simulink model "current_controller_AC"  (R2022a)
settings: Solver=FixedStepAuto  StartTime=0.0  StopTime=0.6  FixedStep=3e-8  RelTol=1e-3
values from neighbouring files (symbols this model uses):
  fs = 50*10^3    (= 50000)    [current_controller_parameters.m]
  Kii = 0.0307    [current_controller_parameters.m]
  Kpi = 9.65    [current_controller_parameters.m]
libraries: spsCurrentMeasurementLib x5, spsMosfetLib x4, spsVoltageMeasurementLib x4, spsSeriesRLCBranchLib x3, spsDCVoltageSourceLib x2, simulink x1, spsACVoltageSourceLib x1, spspowerguiLib x1
settings Model: Creator=RTX  LastModifiedBy=RTX

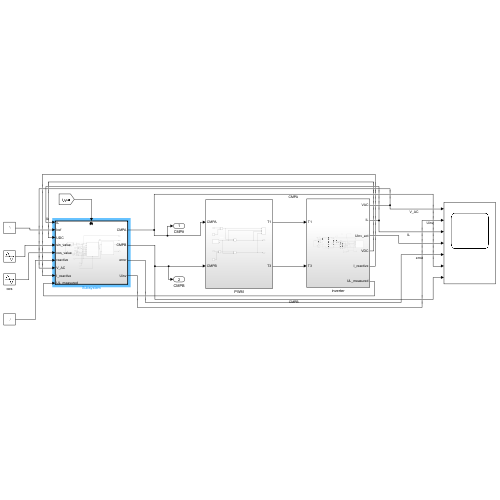
[thumbnail: Simulink's stored preview of the top-level diagram]
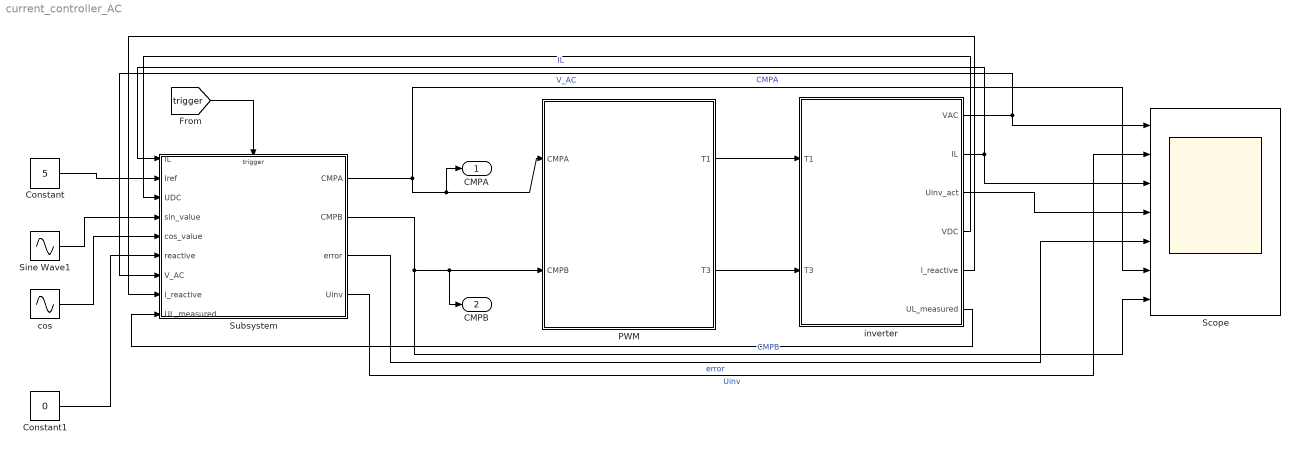
== system current_controller_AC ==
  Constant : Constant  Value=5
  Constant1 : Constant  Value=0
  PWM : Subsystem
  Scope : Scope  NumInputPorts=7
  Sine Wave1 : Sin  Frequency=2*pi*50  SampleTime=0
  Subsystem : Subsystem
  cos : Sin  Frequency=2*pi*50  Phase=pi/2  SampleTime=0
  inverter : Subsystem
  CMPA : Outport
  CMPB : Outport  Port=2
  wires:
  PWM/2(T3) -> inverter/2(T3)
  Subsystem/1(CMPA) -> Scope/6, CMPA/1, PWM/1(CMPA)  "CMPA"
  Constant/1 -> Subsystem/2(Iref)
  [trigger] -> Subsystem/Trigger
  inverter/2(IL) -> Scope/3, Subsystem/1(IL)  "IL"
  inverter/4(VDC) -> Subsystem/3(UDC)
  Sine Wave1/1 -> Subsystem/4(sin_value)
  cos/1 -> Subsystem/5(cos_value)
  Subsystem/2(CMPB) -> Scope/7, CMPB/1, PWM/2(CMPB)  "CMPB"
  PWM/1(T1) -> inverter/1(T1)
  Subsystem/3(error) -> Scope/5  "error"
  inverter/3(Uinv_act) -> Scope/4
  Subsystem/4(Uinv) -> Scope/2  "Uinv"
  inverter/1(VAC) -> Scope/1, Subsystem/7(V_AC)  "V_AC"
  Constant1/1 -> Subsystem/6(reactive)
  inverter/5(I_reactive) -> Subsystem/8(I_reactive)
  inverter/6(UL_measured) -> Subsystem/9(UL_measured)

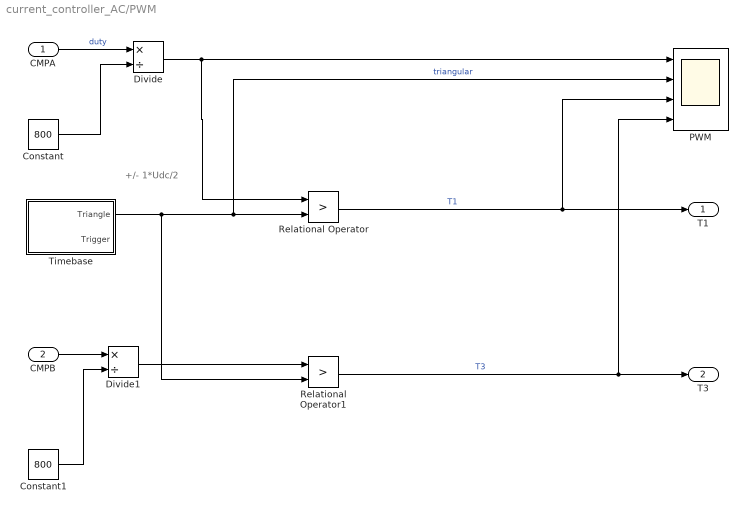
== system current_controller_AC/PWM ==
  note: +/- 1*Udc/2
  CMPA : Inport
  CMPB : Inport  Port=2
  Constant : Constant  Value=800
  Constant1 : Constant  Value=800
  Divide : Product  Inputs=*/
  Divide1 : Product  Inputs=*/
  PWM : Scope  NumInputPorts=4
  Relational Operator : RelationalOperator  Operator=>  OutDataTypeStr=boolean  InputSameDT=off
  Relational Operator1 : RelationalOperator  Operator=>  OutDataTypeStr=boolean  InputSameDT=off
  Timebase : Subsystem
  T1 : Outport
  T3 : Outport  Port=2
  wires:
  Timebase/1(Triangle) -> Relational Operator1/2, Relational Operator/2, PWM/2  "triangular"
  Relational Operator/1 -> T1/1, PWM/3  "T1"
  Relational Operator1/1 -> T3/1, PWM/4  "T3"
  Constant/1 -> Divide/2
  Divide/1 -> Relational Operator/1, PWM/1
  CMPA/1 -> Divide/1  "duty"
  CMPB/1 -> Divide1/1
  Constant1/1 -> Divide1/2
  Divide1/1 -> Relational Operator1/1

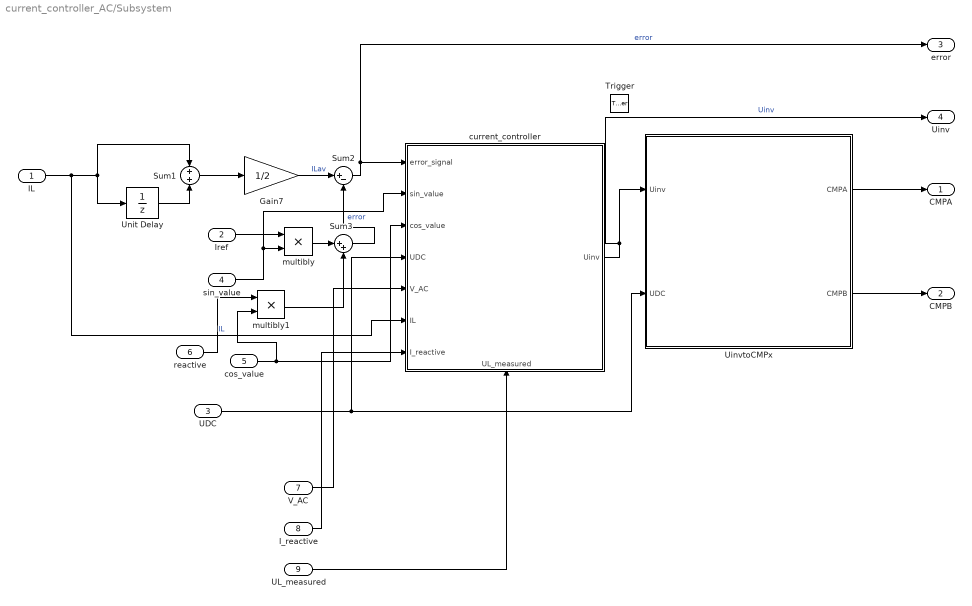
== system current_controller_AC/Subsystem ==
  IL : Inport
  Iref : Inport  Port=2
  UDC : Inport  Port=3
  sin_value : Inport  Port=4
  cos_value : Inport  Port=5
  reactive : Inport  Port=6
  V_AC : Inport  Port=7
  I_reactive : Inport  Port=8
  UL_measured : Inport  Port=9
  Trigger : TriggerPort  TriggerType=either  VariantControl=(inherit)
  Gain7 : Gain  Gain=1/2
  Sum1 : Sum  Inputs=+|+
  Sum2 : Sum  Inputs=|+-
  Sum3 : Sum  Inputs=|++
  UinvtoCMPx : Subsystem
  Unit Delay : UnitDelay  SampleTime=-1  HasFrameUpgradeWarning=on
  current_controller : Subsystem
      settings: PortSchema="{\"entries\":[{\"content\":{\"sides\":[{\"content\":{\"connectorIds\":[\"In1\",\"In2\",\"In3\",\"In4\",\"In5\",\"In6\",\"In7\"]},\"type\":\"ConnectorPlacement.EquallySpacedRectSide\",\"uuid\":\"6c1cedd0-1a51-4e1f-9e97-ae5d47dc470e\"},{\"content\":{\"connectorIds\":[\"Out1\"],\"side\":\"RIGHT\"},\"type\":\"ConnectorPlacement.EquallySpacedRectSide\",\"uuid\":\"d3885633-50ec-4f4d-8704-1aaf5180dd60\"},{\"content\":{\"connectorIds\":[],\"side\":\"TOP\"},\"type\":\"ConnectorPlacement.EquallySpacedRectSide\",\"uuid\":\"50eac74c-805e-49ea-adc0-82172a37a2c7\"},{\"content\":{\"connectorIds\":[\"In8\"],\"side\":\"BOTTOM\"},\"type\":\"ConnectorPlacement.EquallySpacedRectSide\",\"uuid\":\"fc348708-956b-4469-95f9-7d36e2b346e5\"}]},\"type\":\"ConnectorPlacement.EquallySpacedConnector\",\"uuid\":\"1b6e2bfe-76cb-4787-b9f1-7d268bdf583c\"}],\"packageUris\":[\"http://schema.mathworks.com/mf0/Connector/R2020b\"],\"version\":\"1.0\"}"
  multibly : Product  Inputs=**
  multibly1 : Product  Inputs=**
  CMPA : Outport
  CMPB : Outport  Port=2
  error : Outport  Port=3
  Uinv : Outport  Port=4
  wires:
  current_controller/1(Uinv) -> Uinv/1, UinvtoCMPx/1(Uinv)  "Uinv"
  cos_value/1 -> multibly1/2, current_controller/3(cos_value)
  sin_value/1 -> current_controller/2(sin_value), multibly/2
  UinvtoCMPx/1(CMPA) -> CMPA/1
  UinvtoCMPx/2(CMPB) -> CMPB/1
  Unit Delay/1 -> Sum1/2
  IL/1 -> current_controller/6(IL), Sum1/1, Unit Delay/1  "IL"
  Sum1/1 -> Gain7/1
  Gain7/1 -> Sum2/1  "ILav"
  Sum2/1 -> error/1, current_controller/1(error_signal)  "error"
  Iref/1 -> multibly/1
  UDC/1 -> current_controller/4(UDC), UinvtoCMPx/2(UDC)
  reactive/1 -> multibly1/1
  multibly/1 -> Sum3/1
  multibly1/1 -> Sum3/2
  Sum3/1 -> Sum2/2  "error"
  V_AC/1 -> current_controller/5(V_AC)
  I_reactive/1 -> current_controller/7(I_reactive)
  UL_measured/1 -> current_controller/8(UL_measured)

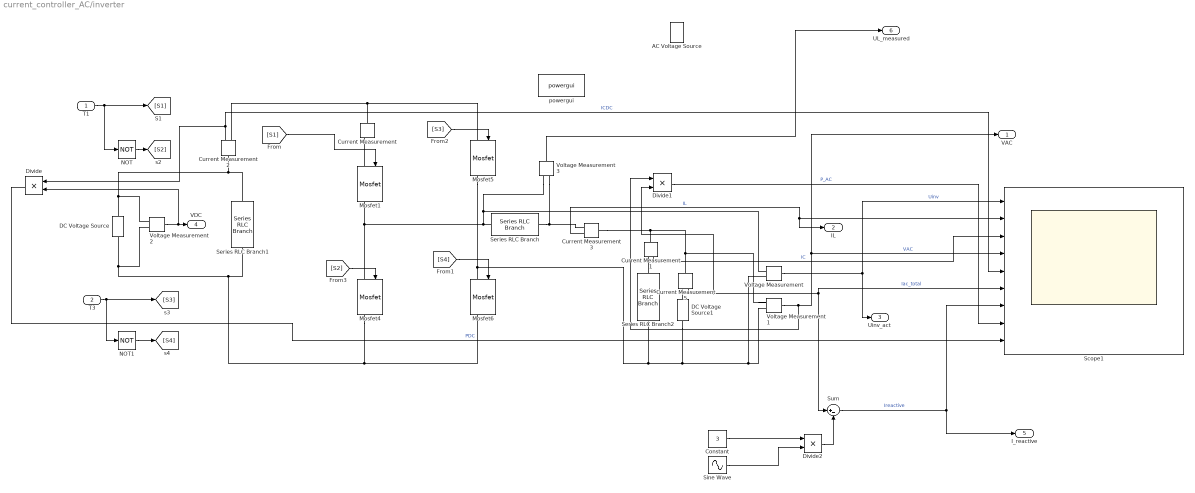
== system current_controller_AC/inverter ==
  T1 : Inport
  T3 : Inport  Port=2
  AC Voltage Source : spsACVoltageSourceLib/AC Voltage Source  Amplitude=48*sqrt(2)  Phase=0  Frequency=50  SampleTime=0  Measurements=None  BusType=swing  Pref=10e3  Qref=0  Qmin=-inf  Qmax=+inf
  Constant : Constant  Value=3
  Current Measurement{,1..3,5} (5 alike) : spsCurrentMeasurementLib/Current Measurement  PhasorSimulation=off  OutputType=Complex  PSBequivalent=0
  DC Voltage Source : spsDCVoltageSourceLib/DC Voltage Source  Amplitude=80  Measurements=None
  DC Voltage Source1 : spsDCVoltageSourceLib/DC Voltage Source  Amplitude=60  Measurements=None
  Divide : Product  Inputs=**
  Divide1 : Product  Inputs=**
  Divide2 : Product  Inputs=**
  Mosfet{1,4..6} (4 alike) : spsMosfetLib/Mosfet  Ron=.1  Lon=0  Rd=.01  Vfd=0  IC=0  Rs=1e5  Cs=inf  Measurements=on
  NOT : Logic  Operator=NOT  IconShape=distinctive  AllPortsSameDT=off  OutDataTypeStr=boolean
  NOT1 : Logic  Operator=NOT  IconShape=distinctive  AllPortsSameDT=off  OutDataTypeStr=boolean
  Scope1 : Scope  NumInputPorts=9
  Series RLC Branch : spsSeriesRLCBranchLib/Series RLC Branch  LConnTagsString=__new0  RConnTagsString=__new0  BranchType=RL  Resistance=0.001  Inductance=600*10^-6  SetiL0=off  InitialCurrent=0  Capacitance=1e-6  Setx0=off  InitialVoltage=0  Measurements=None
  Series RLC Branch1 : spsSeriesRLCBranchLib/Series RLC Branch  LConnTagsString=__new0  RConnTagsString=__new0  BranchType=RC  Resistance=0.001  Inductance=4.06e-3  SetiL0=off  InitialCurrent=0  Capacitance=800e-6  Setx0=on  InitialVoltage=20  Measurements=None
  Series RLC Branch2 : spsSeriesRLCBranchLib/Series RLC Branch  LConnTagsString=__new0  RConnTagsString=__new0  BranchType=RC  Resistance=0.001  Inductance=4.06e-3  SetiL0=off  InitialCurrent=0  Capacitance=16e-6  Setx0=on  InitialVoltage=0  Measurements=None
  Sine Wave : Sin  Frequency=2*pi*50  SampleTime=0
  Sum : Sum  Inputs=|+-
  Voltage Measurement{,1..3} (4 alike) : spsVoltageMeasurementLib/Voltage Measurement  PhasorSimulation=off  OutputType=Complex  PSBequivalent=0
  powergui : spspowerguiLib/powergui  Priority=1  SimulationMode=Continuous  SampleTime=50e-6  frequency=60  Iterations=50  frequencyindice=0  Pbase=100e6  ErrMax=1e-4  UnitsV=kV  UnitsW=MW  buscounter=0  FunctionMessages=off  echomessages=off  EnableUseOfTLC=off  CurrentSourceSwitches=off  DisableSnubberDevices=off  DisableRonSwitches=off  DisableVfSwitches=off  DisplayEquations=off  AutomaticDiscreteSolvers=off  SolverType=Tustin/Backward Euler (TBE)  Interpol=off  ExternalGateDelay=off  methode=off  Ts=100  x0status=blocks  SPID=on  SwTol=0  HookPort=off  NonlinearTolerance=1e-4  nMaxIteration=100  ContinueOnMaxIteration=off  RestoreLinks=warning  ResistiveCurrentMeasurement=off  Frange=[0:2:500]  Ylog=off  Xlog=on  ShowGrid=off  save=off  variable=ZData  structure=0  ZoomFFT=off  StartTime=0.0  cycles=1  DisplayStyle=1  fundamental=60  FreqAxis=off  MaxFrequency=1000  frequencyindicesteady=1  RmsSteady=1  display=off
  VAC : Outport
  IL : Outport  Port=2
  Uinv_act : Outport  Port=3
  VDC : Outport  Port=4
  I_reactive : Outport  Port=5
  UL_measured : Outport  Port=6
  wires:
  Current Measurement3/1 -> IL/1, Scope1/2  "IL"
  Current Measurement2/1 -> Divide/1, Scope1/5  "ICDC"
  [S4] -> Mosfet6/1
  Voltage Measurement/1 -> Scope1/1, Uinv_act/1  "Uinv"
  Current Measurement1/1 -> Scope1/3  "IC"
  [S2] -> Mosfet4/1
  [S3] -> Mosfet5/1
  [S1] -> Mosfet1/1
  T3/1 -> [S3], NOT1/1
  T1/1 -> [S1], NOT/1
  NOT1/1 -> [S4]
  NOT/1 -> [S2]
  Voltage Measurement1/1 -> Divide1/1, VAC/1, Scope1/4  "VAC"
  Voltage Measurement2/1 -> Divide/2, VDC/1
  Divide1/1 -> Scope1/8  "P_AC"
  Current Measurement5/1 -> Divide1/2, Scope1/6, Sum/1  "Iac_total"
  Constant/1 -> Divide2/1
  Sine Wave/1 -> Divide2/2
  Divide2/1 -> Sum/2
  Sum/1 -> I_reactive/1, Scope1/7  "Ireactive"
  Voltage Measurement3/1 -> UL_measured/1
  Divide/1 -> Scope1/9  "PDC"
  connections:
  Current Measurement1/LConn1 -- Voltage Measurement1/LConn1 -- Current Measurement5/LConn1 -- Current Measurement3/LConn1
  Current Measurement2/RConn1 -- Mosfet5/LConn1 -- Current Measurement/LConn1
  Mosfet4/LConn1 -- Voltage Measurement3/LConn1 -- Voltage Measurement/LConn1 -- Series RLC Branch/LConn1 -- Mosfet1/RConn1
  Series RLC Branch1/LConn1 -- DC Voltage Source/RConn1 -- Voltage Measurement2/LConn1 -- Current Measurement2/LConn1
  Mosfet1/LConn1 -- Current Measurement/RConn1
  Series RLC Branch2/LConn1 -- Current Measurement1/RConn1
  Series RLC Branch/RConn1 -- Voltage Measurement3/LConn2 -- Current Measurement3/RConn1
  Mosfet6/LConn1 -- Mosfet5/RConn1 -- Series RLC Branch2/RConn1 -- DC Voltage Source1/LConn1 -- Voltage Measurement1/LConn2 -- Voltage Measurement/LConn2
  Mosfet6/RConn1 -- Mosfet4/RConn1 -- DC Voltage Source/LConn1 -- Voltage Measurement2/LConn2 -- Series RLC Branch1/RConn1
  DC Voltage Source1/RConn1 -- Current Measurement5/RConn1

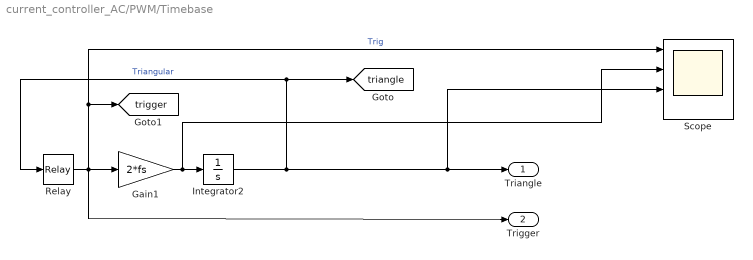
== system current_controller_AC/PWM/Timebase ==
  Gain1 : Gain  Gain=2*fs
  Integrator2 : Integrator  LowerSaturationLimit=0
  Relay : Relay  OnSwitchValue=1  OffSwitchValue=0  OnOutputValue=-1  OffOutputValue=1
  Scope : Scope  NumInputPorts=4
  Triangle : Outport  VectorParamsAs1DForOutWhenUnconnected=off
  Trigger : Outport  Port=2  VectorParamsAs1DForOutWhenUnconnected=off
  tag scope: triangle=global, trigger=global
  wires:
  Integrator2/1 -> Scope/3, Triangle/1, [triangle], Relay/1  "Triangular"
  Relay/1 -> Gain1/1, [trigger], Scope/1, Trigger/1  "Trig"
  Gain1/1 -> Scope/2, Integrator2/1

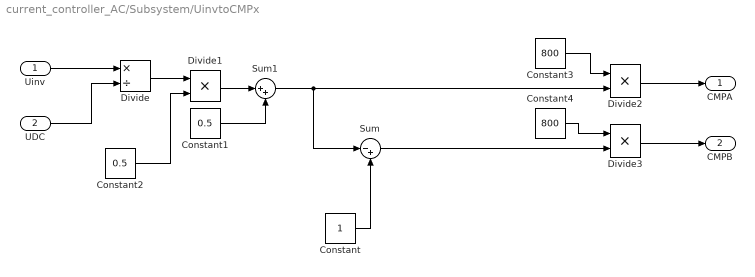
== system current_controller_AC/Subsystem/UinvtoCMPx ==
  Uinv : Inport
  UDC : Inport  Port=2
  Constant : Constant
  Constant1 : Constant  Value=0.5
  Constant2 : Constant  Value=0.5
  Constant3 : Constant  Value=800
  Constant4 : Constant  Value=800
  Divide : Product  Inputs=*/
  Divide1 : Product  Inputs=**
  Divide2 : Product  Inputs=**
  Divide3 : Product  Inputs=**
  Sum : Sum  Inputs=|-+
  Sum1 : Sum  Inputs=|++
  CMPA : Outport
  CMPB : Outport  Port=2
  wires:
  Divide2/1 -> CMPA/1
  Sum/1 -> Divide3/2
  Constant/1 -> Sum/2
  Uinv/1 -> Divide/1
  UDC/1 -> Divide/2
  Divide/1 -> Divide1/1
  Constant2/1 -> Divide1/2
  Divide1/1 -> Sum1/1
  Constant1/1 -> Sum1/2
  Sum1/1 -> Sum/1, Divide2/2
  Constant3/1 -> Divide2/1
  Constant4/1 -> Divide3/1
  Divide3/1 -> CMPB/1

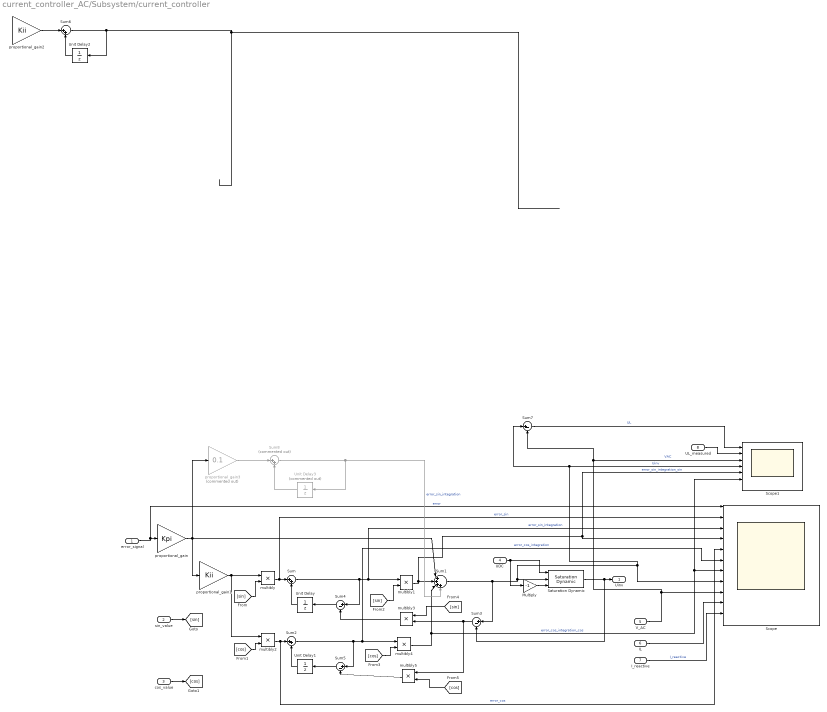
== system current_controller_AC/Subsystem/current_controller ==
  error_signal : Inport
  sin_value : Inport  Port=2
  cos_value : Inport  Port=3
  UDC : Inport  Port=4
  V_AC : Inport  Port=5
  IL : Inport  Port=6
  I_reactive : Inport  Port=7
  UL_measured : Inport  Port=8
  Multiply : Gain  Gain=-1
  Saturation Dynamic : simulink/Discontinuities/Saturation Dynamic  OutMin=[]  OutMax=[]  OutDataTypeStr=Inherit: Same as second input  OutDataType=fixdt(1, 16)  OutScaling=2^-10  DoSatur=off
  Scope : Scope  NumInputPorts=12
  Scope1 : Scope  NumInputPorts=7
  Sum : Sum  Inputs=|++
  Sum1 : Sum  Inputs=|++++
  Sum2 : Sum  Inputs=|++
  Sum{3..5,7} (4 alike) : Sum  Inputs=|+-
  Sum6 : Sum  Inputs=|++
  Sum8 : Sum  Commented=on  Inputs=|++
  Unit Delay : UnitDelay  SampleTime=-1  HasFrameUpgradeWarning=on
  Unit Delay1 : UnitDelay  SampleTime=-1  HasFrameUpgradeWarning=on
  Unit Delay2 : UnitDelay  SampleTime=-1  HasFrameUpgradeWarning=on
  Unit Delay3 : UnitDelay  Commented=on  SampleTime=-1  HasFrameUpgradeWarning=on
  multibly{,1..5} (6 alike) : Product  Inputs=**
  proportional_gain : Gain  Gain=Kpi
  proportional_gain1 : Gain  Gain=Kii
  proportional_gain2 : Gain  Gain=Kii
  proportional_gain3 : Gain  Commented=on  Gain=0.1
  Uinv : Outport
  wires:
  proportional_gain/1 -> proportional_gain3/1, Sum1/1, proportional_gain1/1
  Saturation Dynamic/1 -> Sum3/2, Uinv/1
  error_signal/1 -> Scope/1, proportional_gain/1  "error"
  Sum2/1 -> Sum5/1, Scope/6, multibly4/1  "error_cos_integration"
  [cos] -> multibly4/2
  multibly5/1 -> Sum5/2
  [cos] -> multibly2/2
  multibly/1 -> Scope/2, Sum/1  "error_sin"
  Unit Delay/1 -> Sum/2
  Sum4/1 -> Unit Delay/1
  multibly4/1 -> Scope1/6, Scope/7, Sum1/3  "error_cos_integration_cos"
  [sin] -> multibly/2
  Sum3/1 -> multibly5/1, multibly3/2
  Unit Delay1/1 -> Sum2/2
  Sum/1 -> Sum4/1, Scope/3, multibly1/1  "error_sin_integration"
  sin_value/1 -> [sin]
  proportional_gain1/1 -> multibly2/1, multibly/1
  Sum1/1 -> Sum3/1, Saturation Dynamic/2, Scope/8, Scope1/4, Sum7/1  "Uinv"
  multibly2/1 -> Scope/5, Sum2/1  "error_cos"
  Sum5/1 -> Unit Delay1/1
  multibly3/1 -> Sum4/2
  [cos] -> multibly5/2
  [sin] -> multibly3/1
  cos_value/1 -> [cos]
  [sin] -> multibly1/2
  multibly1/1 -> Scope/4, Scope1/5, Sum1/2  "error_sin_integration_sin"
  UDC/1 -> Saturation Dynamic/1, Multiply/1
  Multiply/1 -> Saturation Dynamic/3
  V_AC/1 -> Sum7/2, Scope1/3, Scope/9  "VAC"
  IL/1 -> Scope/10
  I_reactive/1 -> Scope/11  "I_reactive"
  Sum7/1 -> Scope1/1  "UL"
  UL_measured/1 -> Scope1/2
  Sum6/1 -> Unit Delay2/1
  proportional_gain2/1 -> Sum6/1
  Unit Delay2/1 -> Sum6/2
  ? -> proportional_gain2/1
  proportional_gain3/1 -> Sum8/1
  Unit Delay3/1 -> Sum8/2
  Sum8/1 -> Sum1/4, Unit Delay3/1  "error_sin_integration"
